simulink model "mp_rl_load"  (R2021b)
settings: Solver=daessc  StartTime=0.0  StopTime=simlength  MaxStep=Tc  RelTol=1e-3
values from neighbouring files (symbols this model uses):
  A = -R/L    (= -200)    [init_mp_rl_load.m]    (also in init_mp_rl_load_class.m = 0.99)
  Ad = 1 + A*Ts    (= 0.99)    [init_mp_rl_load.m]
  B = 1/L    (= 200)    [init_mp_rl_load.m]    (also in init_mp_rl_load_class.m = 0.01)
  Bd = B*Ts    (= 0.01)    [init_mp_rl_load.m]
  C = 1    [init_mp_rl_load.m]    (also in init_mp_rl_load_class.m)
  iref_a = 50    [init_mp_rl_load.m]
  R = 1    [init_mp_rl_load.m]    (also in init_mp_rl_load_class.m)
  rho = 0    [init_mp_rl_load.m]    (also in init_mp_rl_load_class.m = 0.0001)
  Ts = 1/20e3    (= 5e-05)    [init_mp_rl_load.m]
  udc = 250    [init_mp_rl_load.m]    (also in init_mp_rl_load_class.m)
  w0 = 2*pi*50    (= 314.159265359)    [init_mp_rl_load.m]
libraries: fl_lib x5, nesl_utility x3
settings Model: Creator=dbagn  LastModifiedBy=dbagn
settings SolverCC: AlgebraicLoopSolver=TrustRegion
settings DebuggingCC: SFMachineParentedDataDiag=warning
settings SFSimCC: CustomCodeUndefinedFunction=UseInterfaceOnly

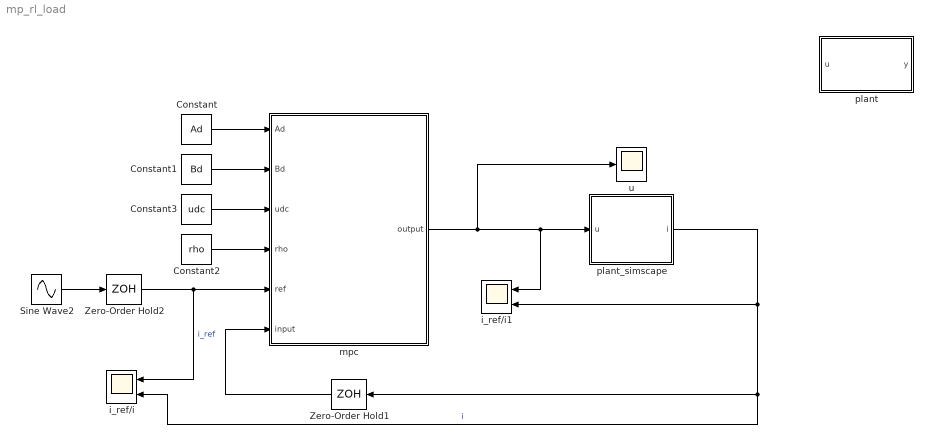
== system mp_rl_load ==
  Constant : Constant  Value=Ad
  Constant1 : Constant  Value=Bd
  Constant2 : Constant  Value=rho
  Constant3 : Constant  Value=udc
  Sine Wave2 : Sin  Amplitude=iref_a  Frequency=w0  SampleTime=0
  Zero-Order Hold1 : ZeroOrderHold  SampleTime=Ts
  Zero-Order Hold2 : ZeroOrderHold  SampleTime=Ts
  i_ref/i : Scope  NumInputPorts=2
  i_ref/i1 : Scope  NumInputPorts=2
  mpc : MATLAB Function  TreatAsAtomicUnit=on  SystemSampleTime=Ts
  "plant " : Subsystem
  plant_simscape : Subsystem
  u : Scope
  wires:
  mpc/1(output) -> plant_simscape/1(u), i_ref/i1/1, u/1
  Sine Wave2/1 -> Zero-Order Hold2/1
  Zero-Order Hold2/1 -> i_ref/i/1, mpc/5(ref)  "i_ref"
  plant_simscape/1(i) -> Zero-Order Hold1/1, i_ref/i/2, i_ref/i1/2  "i"
  Zero-Order Hold1/1 -> mpc/6(input)
  Constant/1 -> mpc/1(Ad)
  Constant1/1 -> mpc/2(Bd)
  Constant2/1 -> mpc/4(rho)
  Constant3/1 -> mpc/3(udc)

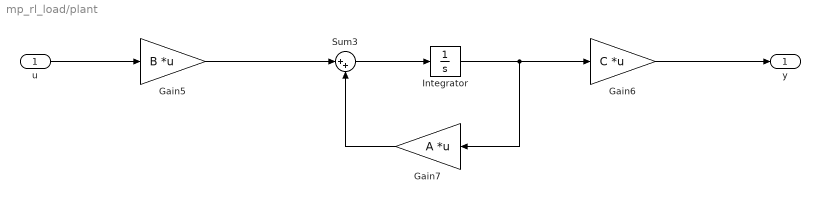
== system mp_rl_load/plant  ==
  u : Inport
  Gain5 : Gain  Gain=B  Multiplication=Matrix(K*u)
  Gain6 : Gain  Gain=C  Multiplication=Matrix(K*u)
  Gain7 : Gain  Gain=A  Multiplication=Matrix(K*u)
  Integrator : Integrator
  Sum3 : Sum  Inputs=|++
  y : Outport
  wires:
  Sum3/1 -> Integrator/1
  Gain7/1 -> Sum3/2
  u/1 -> Gain5/1
  Gain5/1 -> Sum3/1
  Gain6/1 -> y/1
  Integrator/1 -> Gain7/1, Gain6/1

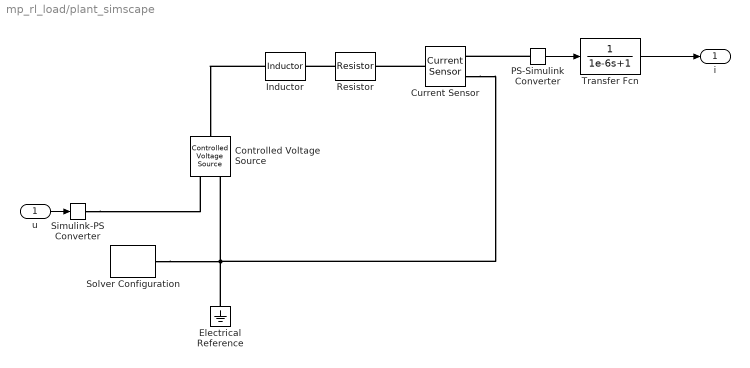
== system mp_rl_load/plant_simscape ==
  u : Inport
  Controlled Voltage Source : fl_lib/Electrical/Electrical Sources/Controlled Voltage Source
  Current Sensor : fl_lib/Electrical/Electrical Sensors/Current Sensor
  Electrical Reference : fl_lib/Electrical/Electrical Elements/Electrical Reference
  Inductor : fl_lib/Electrical/Electrical Elements/Inductor  l=L H  r=0 Ohm  g=1e-9 1/Ohm  i_specify=off  i_priority=None  i=0 A  i_nominal_specify=off  i_nominal_unit=A  i_nominal_value=1  v_specify=off  v_priority=None  v=0 V  v_nominal_specify=off  v_nominal_unit=V  v_nominal_value=1  i_L_specify=off  i_L_priority=High  i_L=0 A  i_L_nominal_specify=off  i_L_nominal_unit=A  i_L_nominal_value=1
  PS-Simulink Converter : nesl_utility/PS-Simulink Converter  PhysicalDomain=network_engine_domain  SubClassName=ps_output  LeftPortType=input  RightPortType=output  PseudoPeriodic=off  Frequencies=[]  Unit=inherit  AffineConversion=off
      settings: SourceProductBaseCode=PW,SS
  Resistor : fl_lib/Electrical/Electrical Elements/Resistor  R=R Ohm  i_specify=off  i_priority=None  i=0 A  i_nominal_specify=off  i_nominal_unit=A  i_nominal_value=1  v_specify=off  v_priority=None  v=0 V  v_nominal_specify=off  v_nominal_unit=V  v_nominal_value=1
  Simulink-PS Converter : nesl_utility/Simulink-PS Converter  PhysicalDomain=network_engine_domain  SubClassName=ps_input  LeftPortType=input  RightPortType=output  PseudoPeriodic=off  Frequencies=[]  NoiseDistribution=none  NoiseParameters=[]  Unit=V  AffineConversion=off  FilteringAndDerivatives=provide  SimscapeFilterOrder=1  InputFilterTimeConstant=0.001  UdotUserProvided=0
      settings: SourceProductBaseCode=PW,SS
  Solver Configuration : nesl_utility/Solver Configuration  PhysicalDomain=network_engine_domain  SubClassName=solver  LeftPortType=input  RightPortType=generic  Tones=[]  Harmonics=[]  SimulateNoise=off  Profile=off  UseLocalSampling=off  EnableSwitchedLinearOptims=on  FrequencyDomain=off  UseCCode=off  RelTol=0.001  AbsTol=1e-06  MinStep=1e-09  ToWorkspace=off  RevertToSquareIcSolve=off  NumHomotopyIterations=100  PhasorMode=off  PhasorModeNumHarmonics=1  DoDC=off  ResidualTolerance=1e-09  UseLocalSolver=on  LocalSolverChoice=NE_BACKWARD_EULER_ADVANCER  LocalSolverSampleTime=Tc  DoFixedCost=on  MaxNonlinIter=3  MaxModeIter=2  ComputeImpulses=off  ImpulseIterations=2  LinearAlgebra=auto  EquationFormulation=NE_TIME_EF  DelaysMemoryBudget=1024  AutomaticFiltering=on  FilteringTimeConstant=0.001  PartitionStorageMethod=AS_NEEDED  PartitionMemoryBudget=1024  PartitionMethod=ROBUST
      settings: SourceProductBaseCode=PW,SS
  Transfer Fcn : TransferFcn  Denominator=[1e-6 1]
  i : Outport
  wires:
  u/1 -> Simulink-PS Converter/1
  PS-Simulink Converter/1 -> Transfer Fcn/1
  Transfer Fcn/1 -> i/1
  connections:
  Simulink-PS Converter/RConn1 -- Controlled Voltage Source/RConn1
  Resistor/LConn1 -- Inductor/RConn1
  Inductor/LConn1 -- Controlled Voltage Source/LConn1
  Electrical Reference/LConn1 -- Current Sensor/RConn2 -- Controlled Voltage Source/RConn2 -- Solver Configuration/RConn1
  Current Sensor/LConn1 -- Resistor/RConn1
  PS-Simulink Converter/LConn1 -- Current Sensor/RConn1

== matlab function mp_rl_load/mpc ==
  data: Ad input; Bd input; udc input; rho input; ref input; input input; output output
function output = mpc(Ad,Bd,udc,rho,ref,input)

    persistent output_z

    if isempty(output_z)
        output_z = 0;
    end
    
    if (output_z == 0)
        
        i_hat_1 = Ad*input+Bd*udc;
        i_hat_2 = Ad*input;
        i_hat_3 = Ad*input-Bd*udc;
        
        J1 = (ref - i_hat_1)^2 + rho*abs(udc-output_z)^2;       % output = 1
        J2 = (ref - i_hat_2)^2 + rho*abs(0-output_z)^2;          % output = 0
        J3 = (ref - i_hat_3)^2 + rho*abs(-udc-output_z)^2;      % output = -1
        
        if ((J1 <= J2) && (J1 <= J3)) 
            output = udc;
        elseif ((J2 <= J1) && (J2 <= J3)) 
            output = 0;
        else 
            output = -udc;
        end 
        
    elseif (output_z == udc)
        
        i_hat_1 = Ad*input+Bd*udc;
        i_hat_2 = Ad*input;
        
        J1 = (ref - i_hat_1)^2 + rho*abs(udc-output_z)^2;       % output = 1
        J2 = (ref - i_hat_2)^2 + rho*abs(0-output_z)^2;          % output = 0
        
        if ((J1 <= J2)) 
            output = udc;
        else
            output = 0;
        end
    else %(output_z == -udc)
        
        i_hat_2 = Ad*input;
        i_hat_3 = Ad*input-Bd*udc;
        
        J2 = (ref - i_hat_2)^2 + rho*abs(0-output_z)^2;          % output = 0
        J3 = (ref - i_hat_3)^2 + rho*abs(-1-output_z)^2;      % output = -1
        
        if ((J2 <= J3)) 
            output = 0;
        else
            output = -udc;
        end
    end
    output_z = output;
end
